simulink model "SDR_audioFile"  (R2022b)
settings: Solver=VariableStepAuto  StartTime=0.0  StopTime=10.0  RelTol=1e-3
libraries: simulink x5, dspquant2 x2, commdigbbndpm3 x2, dspsrcs4 x2, commchan3 x1, dspsigops x1, dspvision x1
settings Model: Creator=RA  LastModifiedBy=Hp
settings RTWCC: GPUComputeCapability=5.0

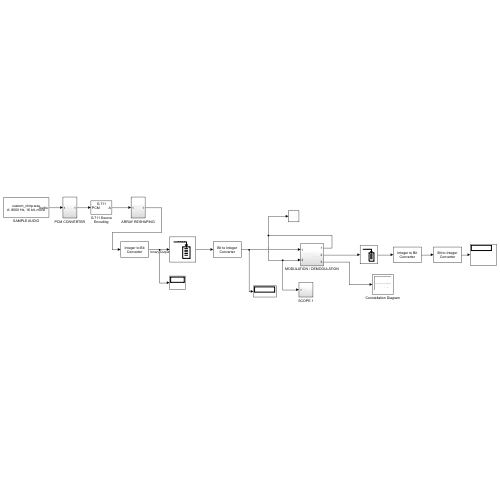
[thumbnail: Simulink's stored preview of the top-level diagram]
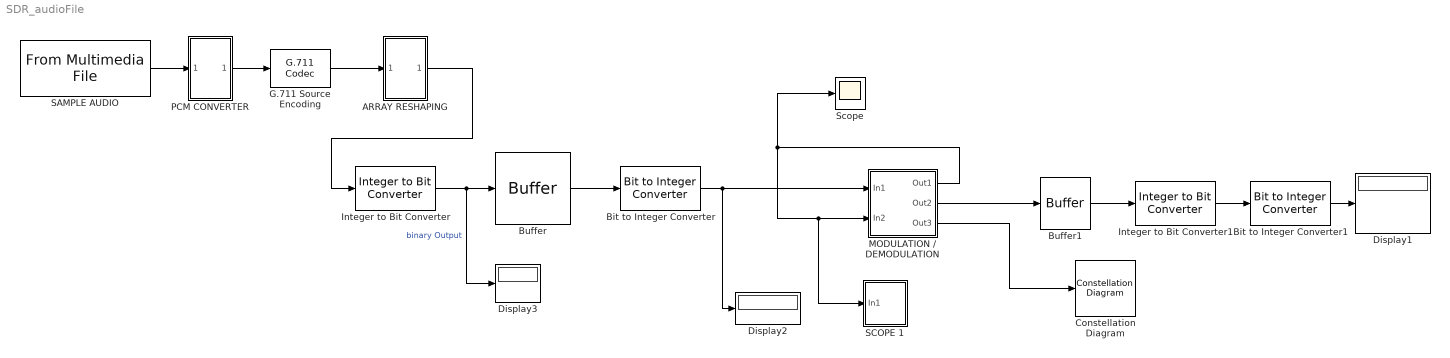
== system SDR_audioFile ==
  ARRAY RESHAPING : Subsystem
  Bit to Integer Converter : simulink/Logic and Bit Operations/Bit to Integer Converter  nbits=2  bitOrder=MSB first  signedOutputValues=Unsigned  outDtype=Inherit via internal rule  outDtypeSigned=Inherit via internal rule
  Bit to Integer Converter1 : simulink/Logic and Bit Operations/Bit to Integer Converter  nbits=8  bitOrder=MSB first  signedOutputValues=Unsigned  outDtype=Inherit via internal rule  outDtypeSigned=Inherit via internal rule
  Buffer : Buffer  N=2  OutputFrames=off
  Buffer1 : Buffer  N=48  OutputFrames=off
  Constellation Diagram : ConstellationDiagram  WindowPosition=[548.000000,46.000000,600.000000,600.000000,]  ScopeFrameLocation=window  SymbolsToDisplaySource=Property  SymbolsToDisplay=1000  XLimits=[-1.46,1.46]  YLimits=[-1.38,1.38]  DefaultConfigurationName=comm.scopes.ConstellationDiagramBlockCfg
  Display1 : Display
  Display2 : Display
  Display3 : Display
  G.711 Source Encoding : dspquant2/G.711 Codec  mode=Encode PCM to A-law  errmode=Warning
  Integer to Bit Converter : simulink/Logic and Bit Operations/Integer to Bit Converter  nbits=8  signedInputValues=Unsigned  bitOrder=MSB first  outDtype=Inherit via internal rule
  Integer to Bit Converter1 : simulink/Logic and Bit Operations/Integer to Bit Converter  nbits=2  signedInputValues=Unsigned  bitOrder=MSB first  outDtype=Inherit via internal rule
  MODULATION / DEMODULATION : Subsystem
  PCM CONVERTER : Subsystem
  SAMPLE AUDIO : dspvision/From Multimedia File  inputFilename=E:\BEE - 13 (B) Semesters\6th Semester(29 Jan 24 -)\Projects\Digital Signal Processing\Simulink Stuff\custom_chirp.wav  readRange=[1 Inf]  loop=on  numPlays=inf  outputStreams=Audio only  videoDataType=single  audioDataType=double  inheritSampleTime=on  userDefinedSampleTime=1/30  noAudioOutput=off  isIntensityVideo=off  fourcc=RGB  colorVideoFormat=Separate color signals  outputEOF=off  dataOrg=Column-major  audioFrameSize=1  computeAudioFrameSize=off  outSamplingMode=Sample based
      settings: LibrarySourceBlock=audiosources/From Multimedia File
  SCOPE 1 : Subsystem
  Scope : Scope
  wires:
  Integer to Bit Converter/1 -> Display3/1, Buffer/1  "binary Output"
  Buffer/1 -> Bit to Integer Converter/1
  Bit to Integer Converter/1 -> MODULATION / DEMODULATION/1(In1), Display2/1
  Buffer1/1 -> Integer to Bit Converter1/1
  Integer to Bit Converter1/1 -> Bit to Integer Converter1/1
  Bit to Integer Converter1/1 -> Display1/1
  MODULATION / DEMODULATION/1(Out1) -> SCOPE 1/1(In1), MODULATION / DEMODULATION/2(In2), Scope/1
  MODULATION / DEMODULATION/2(Out2) -> Buffer1/1
  MODULATION / DEMODULATION/3(Out3) -> Constellation Diagram/1
  ARRAY RESHAPING/1(Out1) -> Integer to Bit Converter/1
  SAMPLE AUDIO/1 -> PCM CONVERTER/1(In1)
  PCM CONVERTER/1(Out1) -> G.711 Source Encoding/1
  G.711 Source Encoding/1 -> ARRAY RESHAPING/1(Inport)

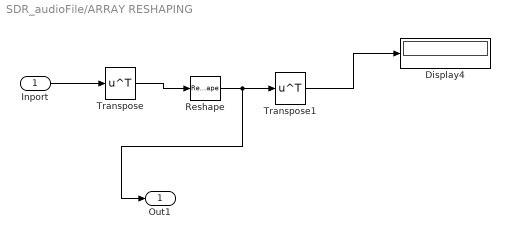
== system SDR_audioFile/ARRAY RESHAPING ==
  Inport : Inport
  Display4 : Display
  Reshape : Reshape
  Transpose : Math  Operator=transpose
  Transpose1 : Math  Operator=transpose
  Out1 : Outport
  wires:
  Transpose/1 -> Reshape/1
  Reshape/1 -> Out1/1, Transpose1/1
  Transpose1/1 -> Display4/1
  Inport/1 -> Transpose/1

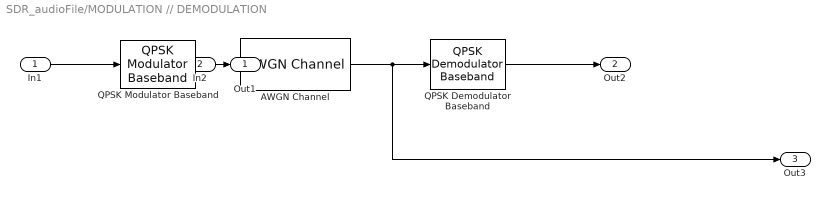
== system SDR_audioFile/MODULATION // DEMODULATION ==
  In1 : Inport
  In2 : Inport  Port=2
  AWGN Channel : commchan3/AWGN Channel  InputProcessing=Columns as channels (frame based)  seed=67  noiseMode="Signal to noise ratio  (SNR)"  EbNodB=10  EsNodB=10  SNRdB=10  bitsPerSym=1  Ps=1  Tsym=(1.000000e-04 * 1)  variance=1
  QPSK Demodulator Baseband : commdigbbndpm3/QPSK Demodulator Baseband  OutType=Integer  DecType=Hard decision  VarSource=Dialog  Variance=1  Dec=Gray  Ph=pi/4  outDtype1=Inherit via internal rule  outDtype2=Inherit via internal rule  derotateFactorWordLen=16  derotateFactorDataTypeStr=Inherit: Same word length as input  derotateFactorLastDataTypeStr=Inherit: Same word length as input
  QPSK Modulator Baseband : commdigbbndpm3/QPSK Modulator Baseband  InType=Integer  Enc=Gray  Ph=pi/4  outDtype=double  outWordLen=16  outUDDataType=sfix(16)  outFracLenMode=Best precision  outFracLen=15  outDataTypeStr=double  outLastDataTypeStr=double
  Out1 : Outport
  Out2 : Outport  Port=2
  Out3 : Outport  Port=3
  wires:
  AWGN Channel/1 -> Out3/1, QPSK Demodulator Baseband/1
  In2/1 -> AWGN Channel/1
  QPSK Modulator Baseband/1 -> Out1/1
  QPSK Demodulator Baseband/1 -> Out2/1
  In1/1 -> QPSK Modulator Baseband/1

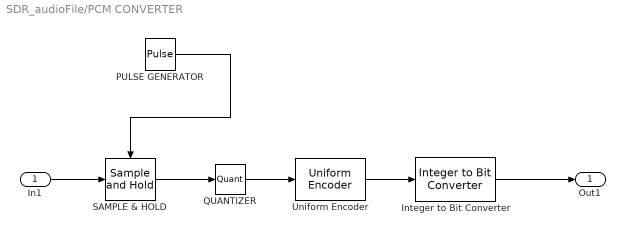
== system SDR_audioFile/PCM CONVERTER ==
  In1 : Inport
  Integer to Bit Converter : simulink/Logic and Bit Operations/Integer to Bit Converter  nbits=16  signedInputValues=Unsigned  bitOrder=MSB first  outDtype=Inherit via internal rule
      settings: LibrarySourceBlock=|
      | commutil2/Integer to Bit
      | Converter
  PULSE GENERATOR : DiscretePulseGenerator  PulseType=Time based  Period=1/18000  PulseWidth=50
  QUANTIZER : Quantizer  QuantizationInterval=1
  SAMPLE & HOLD : dspsigops/Sample and Hold  trig=Rising edge  initCond=0  latchinput=off
  Uniform Encoder : dspquant2/Uniform Encoder  peak=5  bits=16  otype=Unsigned integer
  Out1 : Outport
  wires:
  PULSE GENERATOR/1 -> SAMPLE & HOLD/Trigger
  Uniform Encoder/1 -> Integer to Bit Converter/1
  QUANTIZER/1 -> Uniform Encoder/1
  Integer to Bit Converter/1 -> Out1/1
  SAMPLE & HOLD/1 -> QUANTIZER/1
  In1/1 -> SAMPLE & HOLD/1

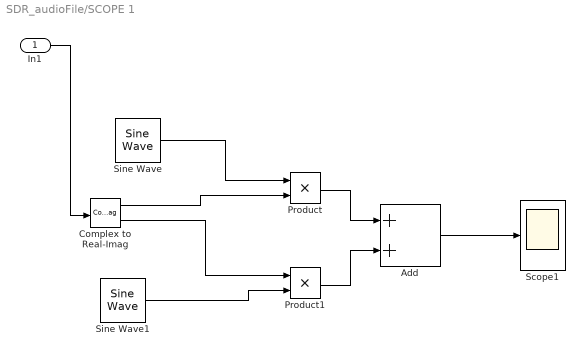
== system SDR_audioFile/SCOPE 1 ==
  In1 : Inport
  Add : Sum
  Complex to Real-Imag : ComplexToRealImag
  Product : Product
  Product1 : Product
  Scope1 : Scope
  Sine Wave : dspsrcs4/Sine Wave  Amplitude=1  Frequency=8*pi  Phase=0  SampleMode=Discrete  OutComplex=Real  CompMethod=Trigonometric fcn  TableSize=Speed  SampleTime=1/10000  SamplesPerFrame=1  ResetState=Restart at time zero  OutputFrames=off  dataType=double  wordLen=16  udDataType=sfix(16)  fracBitsMode=Best precision  numFracBits=15  OutDataTypeStr=double  LastOutDataTypeStr=double
  Sine Wave1 : dspsrcs4/Sine Wave  Amplitude=1  Frequency=8*pi  Phase=pi/2  SampleMode=Discrete  OutComplex=Real  CompMethod=Trigonometric fcn  TableSize=Speed  SampleTime=1/10000  SamplesPerFrame=1  ResetState=Restart at time zero  OutputFrames=off  dataType=double  wordLen=16  udDataType=sfix(16)  fracBitsMode=Best precision  numFracBits=15  OutDataTypeStr=double  LastOutDataTypeStr=double
  wires:
  Complex to Real-Imag/2 -> Product1/1
  Product/1 -> Add/1
  Add/1 -> Scope1/1
  Sine Wave1/1 -> Product1/2
  In1/1 -> Complex to Real-Imag/1
  Complex to Real-Imag/1 -> Product/2
  Product1/1 -> Add/2
  Sine Wave/1 -> Product/1
